simulink model "ev_tms_PID"  (R2023a)
settings: Solver=VariableStepAuto  StartTime=0.0  StopTime=600  FixedStep=1  RelTol=1e-3  AbsTol=1e-3
model workspace: external: MATLAB File /Users/rossschrader/Desktop/ML/ME/_Project/_v3/ev_tms_v3_params.m (data not in the file)
undefined symbols (not defined in the file or in its folder): battery_C1_LUT, battery_capacity_LUT, battery_cell_cp, battery_cell_mass, battery_Em_LUT, battery_N_cells, battery_Qe_init, battery_R0_LUT, battery_R1_LUT, battery_SOC_LUT, battery_T_init, battery_temperature_LUT, bulb, cabin_duct_area, cabin_T_init, chiller_area_primary, chiller_N_baffles, chiller_N_tubes, chiller_tube_D, chiller_tube_L, chiller_wall_conductivity, chiller_wall_thickness, compressor_rpm_LUT, condenser_air_area_flow, condenser_air_area_primary, condenser_W, condenser_wall_conductivity, condenser_wall_thickness, coolant_channel_D, coolant_pipe_D, coolant_T_init, coolant_tank_area, coolant_tank_volume, coolant_valve_D_ratio_max, coolant_valve_D_ratio_min, coolant_valve_displacement, coolant_valve_S_max, evaporator_air_area_flow, evaporator_air_area_primary, evaporator_P_target, evaporator_W, evaporator_wall_conductivity, evaporator_wall_thickness, outlet, pump_speed_max, radiator_air_area_flow, radiator_air_area_primary, radiator_W, radiator_wall_conductivity, radiator_wall_thickness, refrigerant_alpha_init, refrigerant_pipe_D
libraries: fl_lib x221, nesl_utility x79, SimscapeFluids_lib x25, LiBatteryElements_lib x16, sdl_lib x3, slpidlib x2, simulink x1, rllib x1, autolibshared x1, SignalEditorBlockLib x1
(part 5 of 7)

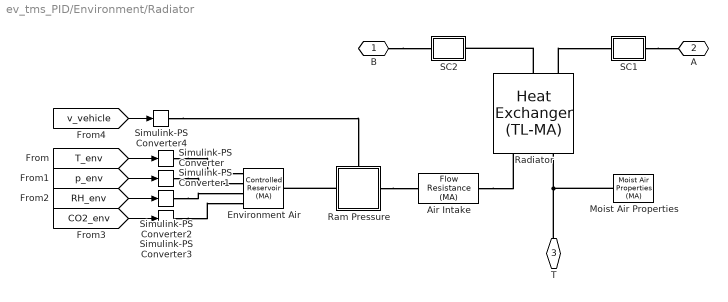
== system ev_tms_PID/Environment/Radiator ==
  Air Intake : fl_lib/Moist Air/Elements/Flow Resistance (MA)  delta_p_nominal=5e-4 MPa  mdot_nominal=1 kg/s  rho_nominal=1.2 kg/m^3  area=cabin_duct_area m^2  laminar_fraction=1e-3
  Environment Air : fl_lib/Moist Air/Elements/Controlled Reservoir (MA)  moisture_spec=foundation.enum.moisture_spec.relative_humidity  trace_gas_spec=foundation.enum.trace_gas_spec.mole_fraction  RH_ws=1  area_A=cabin_duct_area m^2  input_error_spec=foundation.enum.input_range_error.warn
      settings: InternalSimscapePortConfiguration="{\"Bottom\":[],\"Left\":[{\"id\":\"A\",\"label\":\"A\",\"type\":\"foundation.moist_air.moist_air\"}],\"Right\":[{\"id\":\"T\",\"label\":\"T\",\"type\":\"input\"},{\"id\":\"P\",\"label\":\"P\",\"type\":\"input\"},{\"id\":\"W\",\"label\":\"W\",\"type\":\"input\"},{\"id\":\"G\",\"label\":\"G\",\"type\":\"input\"}],\"Top\":[]}"
  Moist Air Properties : fl_lib/Moist Air/Utilities/Moist Air Properties (MA)  R_a=287.047 J/kg/K  T_TLU=[-56.55, -50 : 10 : -10, -5 : 1 : 5, 10 : 10 : 350]' degC  h_a_TLU=[342.416126230579; 349.005511058471; 359.063577249119; 369.119948684177; 379.175469465129; 389.230944678417; 394.258910928084; 395.264534937366; 396.27017101329; 397.275819932805; 398.281482472874; 399.287159410541; 400.292851523015; 401.298559587728; 402.304284382408; 403.310026685143; 404.315787274435; 409.34489180313; 419.404921755863; 429.468036401264; 439.535033154839; 449.606720928652; 459.683919949603; 469.767460521911; 479.858181001348; 489.956925196484; 500.064539372946; 510.181869006204; 520.309755403634; 530.449032296018; 540.60052248087; 550.765034584465; 560.943359995745; 571.136270013102; 581.344513234296; 591.568813210327; 601.809866375885; 612.068340261954; 622.344871990218; 632.640067043998; 642.95449830646; 653.288705353699; 663.643193987949; 674.018435994423; 684.414869104228; 694.832897145098; 705.272890361557; 715.735185886199; 726.220088344236; 736.727870574087; 747.258774447567; 757.813011774199] kJ/kg  mu_a_TLU=[14.2568883320012; 14.6140127728333; 15.1517277055779; 15.6806860159119; 16.2012351072083; 16.7137043125028; 16.9670071730589; 17.017438062815; 17.0677930842452; 17.1180725309876; 17.1682766951315; 17.2184058672268; 17.2684603362935; 17.3184403898301; 17.3683463138234; 17.4181783927569; 17.4679369096204; 17.7156358640698; 18.2056751785154; 18.68879035749; 19.1652344664982; 19.6352478927873; 20.099059103658; 20.5568853601578; 21.0089333871663; 21.4554000014051; 21.8964726992323; 22.3323302062775; 22.7631429910631; 23.1890737447833; 23.6102778293792; 24.0269036959922; 24.4390932757886; 24.8469823450548; 25.2507008663546; 25.6503733074314; 26.0461189394339; 26.4380521159325; 26.8262825340948; 27.2109154792923; 27.5920520543128; 27.969789394274; 28.3442208682439; 28.7154362685068; 29.0835219883356; 29.4485611890712; 29.8106339572472; 30.1698174524429; 30.5261860464955; 30.8798114546565; 31.2307628592324; 31.5791070262086] s*uPa  k_a_TLU=[19.8808489374933; 20.4162454629695; 21.2248743590758; 22.0232452890903; 22.8117314495857; 23.5906913619588; 23.9767075412237; 24.053639990175; 24.1304826682191; 24.2072359051629; 24.2839000294007; 24.3604753679152; 24.4369622462801; 24.5133609886625; 24.5896719178249; 24.6658953551279; 24.7420316205333; 25.1214164701832; 25.8738283029331; 26.6180150229276; 27.3542674377332; 28.0828634735341; 28.8040686837224; 29.5181367785657; 30.2253101618423; 30.9258204644224; 31.6198890677835; 32.3077276126633; 32.9895384896798; 33.6655153099498; 34.33584335461; 35.0007000027879; 35.6602551380254; 36.3146715334901; 36.9641052165342; 37.6087058133173; 38.248616874307; 38.8839761815308; 39.5149160384798; 40.1415635435708; 40.7640408480637; 41.3824653993118; 41.9969501701893; 42.6076038755117; 43.2145311762238; 43.8178328720941; 44.4176060836121; 45.013944423749; 45.6069381602018; 46.1966743687041; 46.783237077953; 47.3667074066625] mW/m/K  p_min=1 kPa  p_max=inf MPa  T_min=-56.55 degC  T_max=350 degC  properties_range_check=simscape.enum.assert.action.error  p_atm=0.101325 MPa  T_atm=20 degC  R_w=461.523 J/kg/K  p_ws_TLU=[1.71168953425982e-06; 3.93770601979424e-06; 1.28411717710344e-05; 3.80051394873809e-05; .00010323902900209; .000259873810798063; .000401741022116384; .000437454836117844; .000476040820618202; .000517704666185737; .000562664883741207; .000611212677444345; .000657088049117899; .000705987905898279; .000758082381149132; .000813549384183233; .000872574861129522; .00122818386934022; .0023392147667769; .00424668834054807; .00738442748706953; .0123512704340234; .0199458019246787; .0312006356960619; .0474147199263783; .0701823607447713; .10141797792131; .143375967241115; .198665399739302; .270259606559999; .361500961984849; .476101381081492; .618139196722055; .792053183687694; 1.0026345688121; 1.25501792086105; 1.55467186826983; 1.90739066433297; 2.31928772772542; 2.79679245576864; 3.34665187151016; 3.97593907083533; 4.69207105435535; 5.5028394740883; 6.41645928168037; 7.4416425436169; 8.58770832955728; 9.86474556030261; 11.2838558865497; 12.8575218898034; 14.6001810568052; 16.5291642526045] MPa  h_w_vap_TLU=[2836.88241275372; 2837.81392500514; 2838.63937175807; 2838.7309929628; 2838.06905313927; 2836.62597341095; 2835.60023952573; 2835.37006381376; 2835.13143158077; 2834.88429145066; 2834.62859062897; 2500.93420564316; 2498.55329907119; 2496.17495082036; 2493.79885912205; 2491.42474723191; 2489.05236104642; 2477.20875029194; 2453.54955988604; 2429.83856603313; 2406.00136954922; 2381.97406342174; 2357.69101156389; 2333.08088387814; 2308.06565480412; 2282.56034405021; 2256.47287422313; 2229.70428017508; 2202.14968030993; 2173.69998896199; 2144.24368406447; 2113.66758247452; 2081.85585110571; 2048.68725710494; 2014.03141249899; 1977.7449923284; 1939.66849592886; 1899.62342931686; 1857.40930169838; 1812.79975416601; 1765.53721731251; 1715.32525772152; 1661.81700477787; 1604.59703745016; 1543.1534616334; 1476.83692476464; 1404.80240352424; 1325.92091736114; 1238.61667822208; 1140.5102987018; 1027.62017777647; 892.733785613825] kJ/kg  h_w_TLU=[2396.55944251649; 2408.68643343608; 2427.1988031141; 2445.702165897; 2464.18429108356; 2482.62529466839; 2491.82135326629; 2493.6580151792; 2495.49372578218; 2497.32843835745; 2499.16210446923; 2500.99462758899; 2502.83092214066; 2504.6665223621; 2506.50140563013; 2508.335548891; 2510.16892865793; 2519.32352241995; 2537.56068088674; 2555.67742615292; 2573.6403223998; 2591.4109179101; 2608.9455037701; 2626.19492016262; 2643.10444358428; 2659.61377634497; 2675.58278696023; 2696.1846256545; 2716.49989553741; 2736.6235210957; 2756.61216047011; 2776.50561773853; 2796.33378922508; 2816.11979583049; 2835.88181423877; 2855.63430574511; 2875.38889327595; 2895.15500577172; 2914.94035964689; 2934.75132290228; 2954.59319330244; 2974.47041285505; 2994.38673458964; 3014.34535328009; 3034.34900867103; 3054.40006755764; 3074.50058946898; 3094.65237953784; 3114.85703128106; 3135.11596137801; 3155.43043805905; 3175.80160435813] kJ/kg  mu_w_TLU=[6.81365662228272; 7.04953750742707; 7.40970098298307; 7.76991278093907; 8.13017290129507; 8.49048134405107; 8.67065368632907; 8.70668960445667; 8.74272600580827; 8.77876289038387; 8.81480025818347; 8.85083810920707; 8.88687644345467; 8.92291526092627; 8.95895456162187; 8.99499434554147; 9.03103461268507; 9.21124319676307; 9.57169660671907; 9.93219833907507; 10.2927483938311; 10.6533467709871; 11.0139934705431; 11.3746884924991; 11.7354318368551; 12.0962235036111; 12.4570634927671; 12.8179518043231; 13.1788884382791; 13.5398733946351; 13.9009066733911; 14.2619882745471; 14.6231181981031; 14.9842964440591; 15.3455230124151; 15.7067979031711; 16.0681211163271; 16.4294926518831; 16.7909125098391; 17.1523806901951; 17.5138971929511; 17.8754620181071; 18.2370751656631; 18.5987366356191; 18.9604464279751; 19.3222045427311; 19.6840109798871; 20.0458657394431; 20.4077688213991; 20.7697202257551; 21.1317199525111; 21.4937680016671] s*uPa  k_w_TLU=[11.46288215976; 11.941997488935; 12.676358586935; 13.414208884935; 14.155548382935; 14.900377080935; 15.274099879935; 15.348949115735; 15.423833243535; 15.498752263335; 15.573706175135; 15.648694978935; 15.723718674735; 15.798777262535; 15.873870742335; 15.948999114135; 16.024162377935; 16.400502076935; 17.155798374935; 17.914583872935; 18.676858570935; 19.442622468935; 20.211875566935; 20.984617864935; 21.760849362935; 22.540570060935; 23.323779958935; 24.110479056935; 24.900667354935; 25.694344852935; 26.491511550935; 27.292167448935; 28.096312546935; 28.903946844935; 29.715070342935; 30.529683040935; 31.347784938935; 32.169376036935; 32.994456334935; 33.823025832935; 34.655084530935; 35.490632428935; 36.329669526935; 37.172195824935; 38.018211322935; 38.867716020935; 39.720709918935; 40.577193016935; 41.437165314935; 42.300626812935; 43.167577510935; 44.038017408935] mW/m/K  D_w=25 mm^2/s  trace_gas_model=foundation.enum.trace_gas_model.track_fraction  R_g=188.923 J/kg/K  h_g_TLU=[439.555216260064; 444.670268200251; 452.538618847003; 460.487124258496; 468.522588768941; 476.649415958793; 480.74798538725; 481.57054318762; 482.394052398751; 483.218514288831; 484.043930029015; 484.870300696555; 485.697627277859; 486.525910671489; 487.355151691079; 488.185351068185; 489.016509455051; 493.186704139431; 501.599194953048; 510.107689961685; 518.711611080182; 527.410026793075; 536.201764778798; 545.085474203452; 554.059675505208; 563.122805485367; 572.27325096919; 581.509373027928; 590.829525105886; 600.232066705818; 609.715373581392; 619.277845178105; 628.917909922924; 638.634028838794; 648.424697859328; 658.288449140109; 668.223851601449; 678.229510889093; 688.304068901113; 698.44620299875; 708.654624994591; 718.928079991818; 729.265345132425; 739.665228299475; 750.126566808087; 760.648226111439; 771.229098541268; 781.868102096908; 792.564179292476; 803.316296068366; 814.123440770426; 824.984623198037] kJ/kg  mu_g_TLU=[10.8921054191698; 11.2215357085649; 11.7233300740382; 12.2234238147811; 12.7215124453467; 13.2173328890673; 13.4643203184773; 13.5136406274989; 13.562934752385; 13.6122025024997; 13.6614436900741; 13.7106581301692; 13.7598456406398; 13.8090060420983; 13.8581391578796; 13.9072448140062; 13.9563228391538; 14.2012926853717; 14.6890687376044; 15.1738428124161; 15.6554929043332; 16.1339159800463; 16.6090257998657; 17.0807510097148; 17.5490334645512; 18.0138267508952; 18.4750948814453; 18.9328111390399; 19.3869570507278; 19.8375214755778; 20.2844997922255; 20.7278931741254; 21.1677079421287; 21.6039549853963; 22.036649242835; 22.4658092382469; 22.8914566632375; 23.3136160026627; 23.7323141980278; 24.1475803447965; 24.5594454200432; 24.9679420372927; 25.3731042257492; 25.774967231431; 26.1735673380029; 26.5689417053362; 26.9611282240413; 27.350165384404; 27.73609215832; 28.118947892972; 28.4987722151178; 28.8756049449796] s*uPa  k_g_TLU=[10.489430678843; 10.9507672150864; 11.666197960308; 12.392559739764; 13.1299519771612; 13.8778409888416; 14.2554325416312; 14.3312274189707; 14.4071122346908; 14.4830860227061; 14.5591478179508; 14.6352966574703; 14.7115315815553; 14.787851634907; 14.8642558678259; 14.9407433374142; 15.0173131087819; 15.401364480906; 16.1751373988038; 16.9558134611595; 17.7432208682398; 18.5366976599676; 19.3360988502003; 20.1412225692689; 20.9517507672929; 21.7672310558863; 22.5871115634685; 23.4107980865695; 24.2377021890869; 25.0672663781241; 25.8989689893876; 26.732318357514; 27.5668446164644; 28.4020933015927; 29.2376215872816; 30.0729965057542; 30.9077942826816; 31.7416001931033; 32.5740086297993; 33.4046232539953; 34.2330571812868; 35.0589331874899; 35.8818839295189; 36.701552179391; 37.5175910702657; 38.3296643536716; 39.1374466671854; 39.9406238119064; 40.7388930391313; 41.5319633456945; 42.3195557774861; 43.1014037407076] mW/m/K  D_g=16 mm^2/s
  Radiator : SimscapeFluids_lib/Fluid Network Interfaces/Heat Exchangers/Heat Exchanger (TL-MA)  flow_arrangement=fluids.interfaces.heat_exchangers.enum.FlowArrangementTLMA.Cross  cross_flow_arrangement=fluids.interfaces.heat_exchangers.enum.CrossFlowArrangementTLMA.MixedUnmixed  R_wall=radiator_wall_thickness / radiator_air_area_primary / radiator_wall_conductivity K/kW  area_A1=pi * coolant_pipe_D^2 / 4 m^2  area_B1=pi * coolant_pipe_D^2 / 4 m^2  area_A2=cabin_duct_area m^2  area_B2=cabin_duct_area m^2  flow_geometry_TL=fluids.interfaces.heat_exchangers.enum.FlowGeometryTL.InsideTubes  tube_num_TL=radiator_N_tubes  tube_length_TL=radiator_L m  tube_cross_section_TL=fluids.interfaces.heat_exchangers.enum.TubeCrossSection.Rectangular  tube_diameter_TL=0.1 m  tube_width_TL=radiator_W m  tube_height_TL=radiator_tube_H m  tube_inner_diameter_TL=0.05 m  tube_outer_diameter_TL=0.1 m  tube_flow_area_TL=0.01 m^2  tube_wetted_perimeter_TL=0.4 m  tube_heat_perimeter_TL=0.4 m  tube_pressure_loss_spec_TL=fluids.interfaces.heat_exchangers.enum.TubePressureLossSpec.Haaland  tube_loss_coeff_TL=10  tube_local_pressure_loss_spec_TL=fluids.thermal_liquid.pipes_fittings.enum.LocalLossSpec.AggregateLength  tube_length_add_TL=radiator_tube_Leq m  tube_local_loss_coefficient_TL=0.1  tube_roughness_pressure_TL=15e-6 m  tube_Re_lam_pressure_TL=2000  tube_Re_tur_pressure_TL=4000  tube_shape_factor_generic_TL=64  tube_heat_coeff_spec_TL=fluids.interfaces.heat_exchangers.enum.TubeHeatCoeffSpec.Gneilinski  tube_colburn_coeff_TL=[.023, .8, .33]  tube_roughness_heat_TL=15e-6 m  tube_Re_lam_heat_TL=2000  tube_Re_tur_heat_TL=4000  tube_Nu_lam_generic_TL=3.66  bank_arrangement_TL=fluids.interfaces.heat_exchangers.enum.BankArrangement.Inline  bank_num_rows_TL=5  bank_tubes_per_row_TL=5  bank_width_TL=1 m  bank_tube_diameter_TL=0.05 m  bank_longitudinal_pitch_TL=0.15 m  bank_transverse_pitch_TL=0.15 m  bank_pressure_loss_spec_TL=fluids.interfaces.heat_exchangers.enum.BankPressureLossSpec.Martin  bank_euler_TL=10  bank_heat_coeff_spec_TL=fluids.interfaces.heat_exchangers.enum.BankHeatCoeffSpec.Martin  bank_colburn_coeff_TL=[.27, .63, .36]  generic_flow_area_TL=0.01 m^2  generic_heat_area_TL=2 m^2  generic_volume_TL=0.05 m^3  generic_loss_coeff_TL=10  generic_colburn_coeff_TL=[.023, .8, .33]  fouling_factor_TL=0.1 m^2*K/kW  fin_area_TL=0 m^2  fin_efficiency_TL=0  p_init_TL=coolant_p_init MPa  T_init_TL=coolant_T_init degC  flow_geometry_MA=fluids.interfaces.heat_exchangers.enum.FlowGeometryMA.Generic  tube_num_MA=1  tube_length_MA=5 m  tube_cross_section_MA=fluids.interfaces.heat_exchangers.enum.TubeCrossSection.Circular  tube_diameter_MA=0.1 m  tube_width_MA=0.1 m  tube_height_MA=0.1 m  tube_inner_diameter_MA=0.05 m  tube_outer_diameter_MA=0.1 m  tube_flow_area_MA=0.01 m^2  tube_wetted_perimeter_MA=0.4 m  tube_heat_perimeter_MA=0.4 m  tube_pressure_loss_spec_MA=fluids.interfaces.heat_exchangers.enum.TubePressureLossSpec.Haaland  tube_loss_coeff_MA=10  tube_local_pressure_loss_spec_MA=fluids.moist_air.pipes_fittings.enum.LocalLossSpec.AggregateLength  tube_length_add_MA=0.1 m  tube_local_loss_coefficient_MA=0.1  tube_roughness_pressure_MA=15e-6 m  tube_Re_lam_pressure_MA=2000  tube_Re_tur_pressure_MA=4000  tube_shape_factor_generic_MA=64  tube_heat_coeff_spec_MA=fluids.interfaces.heat_exchangers.enum.TubeHeatCoeffSpec.Gneilinski  tube_colburn_coeff_MA=[.023, .8, .33]  tube_roughness_heat_MA=15e-6 m  tube_Re_lam_heat_MA=2000  tube_Re_tur_heat_MA=4000  tube_Nu_lam_generic_MA=3.66  bank_arrangement_MA=fluids.interfaces.heat_exchangers.enum.BankArrangement.Inline  bank_num_rows_MA=5  bank_tubes_per_row_MA=5  bank_width_MA=1 m  bank_tube_diameter_MA=0.05 m  bank_longitudinal_pitch_MA=0.15 m  bank_transverse_pitch_MA=0.15 m  bank_pressure_loss_spec_MA=fluids.interfaces.heat_exchangers.enum.BankPressureLossSpec.Martin  bank_euler_MA=10  bank_heat_coeff_spec_MA=fluids.interfaces.heat_exchangers.enum.BankHeatCoeffSpec.Martin  bank_colburn_coeff_MA=[.27, .63, .36]  generic_flow_area_MA=radiator_air_area_flow m^2  generic_heat_area_MA=radiator_air_area_primary m^2  generic_volume_MA=radiator_air_area_flow * radiator_W m^3  generic_loss_coeff_MA=10  generic_colburn_coeff_MA=[0.27, 0.63, 0.36]  fouling_factor_MA=0.1 m^2*K/kW  fin_area_MA=radiator_air_area_fins m^2  fin_efficiency_MA=0.7  p_init_MA=cabin_p_init MPa  T_init_MA=cabin_T_init degC  moisture_spec_MA=foundation.enum.moisture_spec.relative_humidity  RH_init_MA=cabin_RH_init  x_w_init_MA=0.01  y_w_init_MA=0.01  HR_init_MA=0.01  trace_gas_spec_MA=foundation.enum.trace_gas_spec.mole_fraction  x_g_init_MA=0.001  y_g_init_MA=cabin_CO2_init  RH_ws_MA=1
      settings: InternalSimscapePortConfiguration="{\"Bottom\":[],\"Left\":[{\"id\":\"A1\",\"label\":\"A1\",\"type\":\"foundation.thermal_liquid.thermal_liquid\"},{\"id\":\"B1\",\"label\":\"B1\",\"type\":\"foundation.thermal_liquid.thermal_liquid\"}],\"Right\":[{\"id\":\"A2\",\"label\":\"A2\",\"type\":\"foundation.moist_air.moist_air\"},{\"id\":\"B2\",\"label\":\"B2\",\"type\":\"foundation.moist_air.moist_air\"}],\"Top\":[{\"id\":\"W\",\"label\":\"W\",\"type\":\"output\"}]}"
  Ram Pressure : Subsystem
      settings: PortSchema="{\"entries\":[{\"content\":{\"sides\":[{\"content\":{\"connectorIds\":[\"LConn1\"]},\"type\":\"ConnectorPlacement.EquallySpacedRectSide\",\"uuid\":\"75e3029b-49fb-4aa2-a270-5647ec8f7cc2\"},{\"content\":{\"connectorIds\":[\"RConn1\"],\"side\":\"RIGHT\"},\"type\":\"ConnectorPlacement.EquallySpacedRectSide\",\"uuid\":\"a5773782-5ea1-4526-866f-91c4aa99dd69\"},{\"content\":{\"connectorIds\":[\"LConn2\"],\"side\":\"TOP\"},\"type\":\"ConnectorPlacement.EquallySpacedRectSide\",\"uuid\":\"b1426a6c-920c-4fe3-a6f1-49137f31d8b5\"}]},\"type\":\"ConnectorPlacement.EquallySpacedConnector\",\"uuid\":\"8a57436c-822b-4551-8b15-f9c616e1048b\"}],\"packageUris\":[\"http://schema.mathworks.com/mf0/Connector/R2020b\"],\"version\":\"1.0\"}"
  SC1 : Subsystem
      mask Display: disp(get_param(gcb, 'Name'))
  SC2 : Subsystem
      mask Display: disp(get_param(gcb, 'Name'))
  Simulink-PS Converter : nesl_utility/Simulink-PS Converter  PhysicalDomain=network_engine_domain  SubClassName=ps_input  LeftPortType=input  RightPortType=output  PseudoPeriodic=off  Frequencies=[]  NoiseDistribution=none  NoiseParameters=[]  Unit=degC  AffineConversion=on  FilteringAndDerivatives=provide  SimscapeFilterOrder=1  InputFilterTimeConstant=0.001  UdotUserProvided=0
  Simulink-PS Converter1 : nesl_utility/Simulink-PS Converter  PhysicalDomain=network_engine_domain  SubClassName=ps_input  LeftPortType=input  RightPortType=output  PseudoPeriodic=off  Frequencies=[]  NoiseDistribution=none  NoiseParameters=[]  Unit=MPa  AffineConversion=off  FilteringAndDerivatives=provide  SimscapeFilterOrder=1  InputFilterTimeConstant=0.001  UdotUserProvided=0
  Simulink-PS Converter2 : nesl_utility/Simulink-PS Converter  PhysicalDomain=network_engine_domain  SubClassName=ps_input  LeftPortType=input  RightPortType=output  PseudoPeriodic=off  Frequencies=[]  NoiseDistribution=none  NoiseParameters=[]  Unit=1  AffineConversion=off  FilteringAndDerivatives=provide  SimscapeFilterOrder=1  InputFilterTimeConstant=0.001  UdotUserProvided=0
  Simulink-PS Converter3 : nesl_utility/Simulink-PS Converter  PhysicalDomain=network_engine_domain  SubClassName=ps_input  LeftPortType=input  RightPortType=output  PseudoPeriodic=off  Frequencies=[]  NoiseDistribution=none  NoiseParameters=[]  Unit=1  AffineConversion=off  FilteringAndDerivatives=provide  SimscapeFilterOrder=1  InputFilterTimeConstant=0.001  UdotUserProvided=0
  Simulink-PS Converter4 : nesl_utility/Simulink-PS Converter  PhysicalDomain=network_engine_domain  SubClassName=ps_input  LeftPortType=input  RightPortType=output  PseudoPeriodic=off  Frequencies=[]  NoiseDistribution=none  NoiseParameters=[]  Unit=km/hr  AffineConversion=off  FilteringAndDerivatives=provide  SimscapeFilterOrder=1  InputFilterTimeConstant=0.001  UdotUserProvided=0
  B : PMIOPort  Side=Left
  A : PMIOPort  Port=2  Side=Right
  T : PMIOPort  Port=3  Side=Right
  wires:
  [RH_env] -> Simulink-PS Converter2/1
  [CO2_env] -> Simulink-PS Converter3/1
  [T_env] -> Simulink-PS Converter/1
  [p_env] -> Simulink-PS Converter1/1
  [v_vehicle] -> Simulink-PS Converter4/1
  connections:
  B/RConn1 -- SC2/LConn1
  Radiator/LConn1 -- SC1/LConn1
  SC1/RConn1 -- A/RConn1
  Radiator/LConn2 -- SC2/RConn1
  Simulink-PS Converter1/RConn1 -- Environment Air/RConn2
  Simulink-PS Converter2/RConn1 -- Environment Air/RConn3
  Simulink-PS Converter3/RConn1 -- Environment Air/RConn4
  Simulink-PS Converter/RConn1 -- Environment Air/RConn1
  T/RConn1 -- Moist Air Properties/RConn1 -- Radiator/RConn1
  Air Intake/RConn1 -- Radiator/RConn2
  Ram Pressure/RConn1 -- Air Intake/LConn1
  Ram Pressure/LConn1 -- Environment Air/LConn1
  Simulink-PS Converter4/RConn1 -- Ram Pressure/LConn2

== system ev_tms_PID/Environment/Radiator Bypass Valve ==
  Bias : Bias  Bias=-1  SaturateOnIntegerOverflow=off
  Flow Resistance (TL) : fl_lib/Thermal Liquid/Elements/Flow Resistance (TL)  delta_p_nominal=0.001 MPa  mdot_nominal=0.3 kg/s  area=pi * coolant_pipe_D^2 / 4 m^2  laminar_fraction=1e-3
  Gain : Gain  Gain=2
  Max Valve Displacement [m] : Gain  Gain=coolant_valve_displacement
  Radiator Bypass Valve : SimscapeFluids_lib/Thermal Liquid/Valves & Orifices/Directional Control Valves/3-Way Directional Valve (TL)  open_orifices_pos=fluids.thermal_liquid.valves.directional_control_valves.enum.OpenOrifices3Way.PA  open_orifices_neg=fluids.thermal_liquid.valves.directional_control_valves.enum.OpenOrifices3Way.AT  area_spec=fluids.thermal_liquid.valves.directional_control_valves.enum.area_spec.identical  valve_spec=fluids.thermal_liquid.valves.enum.orifice_spec.linear  del_S_max=coolant_valve_displacement m  area_max=pi * (coolant_valve_D_ratio_max*coolant_pipe_D)^2 / 4 m^2  del_S_TLU=[0 0.002 0.004 0.007 0.017] m  valve_area_TLU=[1e-09, 2.0352e-07, 4.0736e-05, .00011438, .00034356] m^2  del_S_flow_TLU=[0 0.002 0.004 0.007 0.017] m  p_diff_TLU=[-.1, .3, .5, .7] MPa  vol_flow_TLU=1e-3 * [1.7e-05, 2e-05, 2.6e-05; .0035, .0045, .0053; .7, .9, 1.06; 1.96, 2.5, 3; 6, 7.7, 9.13] m^3/s  mdot_TLU=[-1e-05, 1.7e-05, 2e-05, 2.6e-05; -.002, .0035, .0045, .0053; -.4, .7, .9, 1.06; -1.13, 1.96, 2.5, 3; -3.45, 6, 7.7, 9.13] kg/s  T_ref_in=293.15 K  p_ref_in=0.101325 MPa  area_leak=pi * (coolant_valve_D_ratio_min*coolant_pipe_D)^2 / 4 m^2  Cd=0.7  Re_c=12  smoothing_factor=0.01  pressure_recovery=simscape.enum.onoff.on  area=pi * coolant_pipe_D^2 / 4 m^2  S_max_PA=coolant_valve_S_max m  del_S_max_PA=coolant_valve_displacement-(coolant_valve_displacement)*(pi * (coolant_valve_D_ratio_min*coolant_pipe_D)^2 / 4)/(pi * (coolant_valve_D_ratio_max*coolant_pipe_D)^2 / 4) m  area_max_PA=pi * (coolant_valve_D_ratio_max*coolant_pipe_D)^2 / 4 m^2  del_S_TLU_PA=[0 0.002 0.004 0.007 0.017] m  valve_area_TLU_PA=[1e-09, 2.0352e-07, 4.0736e-05, .00011438, .00034356] m^2  del_S_flow_TLU_PA=[0 0.002 0.004 0.007 0.017] m  p_diff_TLU_PA=[-.1, .3, .5, .7] MPa  vol_flow_TLU_PA=1e-3 * [1.7e-05, 2e-05, 2.6e-05; .0035, .0045, .0053; .7, .9, 1.06; 1.96, 2.5, 3; 6, 7.7, 9.13] m^3/s  mdot_TLU_PA=[-1e-05, 1.7e-05, 2e-05, 2.6e-05; -.002, .0035, .0045, .0053; -.4, .7, .9, 1.06; -1.13, 1.96, 2.5, 3; -3.45, 6, 7.7, 9.13] kg/s  S_max_AT=-coolant_valve_S_max m  del_S_max_AT=coolant_valve_displacement-(coolant_valve_displacement)*(pi * (coolant_valve_D_ratio_min*coolant_pipe_D)^2 / 4)/(pi * (coolant_valve_D_ratio_max*coolant_pipe_D)^2 / 4) m  area_max_AT=pi * (coolant_valve_D_ratio_max*coolant_pipe_D)^2 / 4 m^2  del_S_TLU_AT=[0 0.002 0.004 0.007 0.017] m  valve_area_TLU_AT=[1e-09, 2.0352e-07, 4.0736e-05, .00011438, .00034356] m^2  del_S_flow_TLU_AT=[0 0.002 0.004 0.007 0.017] m  p_diff_TLU_AT=[-.1, .3, .5, .7] MPa  vol_flow_TLU_AT=1e-3 * [1.7e-05, 2e-05, 2.6e-05; .0035, .0045, .0053; .7, .9, 1.06; 1.96, 2.5, 3; 6, 7.7, 9.13] m^3/s  mdot_TLU_AT=[-1e-05, 1.7e-05, 2e-05, 2.6e-05; -.002, .0035, .0045, .0053; -.4, .7, .9, 1.06; -1.13, 1.96, 2.5, 3; -3.45, 6, 7.7, 9.13] kg/s  S_max_PT=2.5e-3 m  del_S_max_PT=0.005 m  area_max_PT=1e-4 m^2  del_S_TLU_PT=[0, .002, .004, .007, .017] m  valve_area_TLU_PT=[1e-09, 2.0352e-07, 4.0736e-05, .00011438, .00034356] m^2  del_S_flow_TLU_PT=[0, .002, .004, .007, .017] m  p_diff_TLU_PT=[.3, .5, .7] MPa  vol_flow_TLU_PT=1e-3 * [1.7e-05, 2e-05, 2.6e-05; .0035, .0045, .0053; .7, .9, 1.06; 1.96, 2.5, 3; 6, 7.7, 9.13] m^3/s  mdot_TLU_PT=[1.7e-05, 2e-05, 2.6e-05; .0035, .0045, .0053; .7, .9, 1.06; 1.96, 2.5, 3; 6, 7.7, 9.13] kg/s
      settings: InternalSimscapePortConfiguration="{\"Bottom\":[],\"Left\":[{\"id\":\"A\",\"label\":\"A\",\"type\":\"foundation.thermal_liquid.thermal_liquid\"}],\"Right\":[{\"id\":\"S\",\"label\":\"S\",\"type\":\"input\"},{\"id\":\"P\",\"label\":\"P\",\"type\":\"foundation.thermal_liquid.thermal_liquid\"},{\"id\":\"T\",\"label\":\"T\",\"type\":\"foundation.thermal_liquid.thermal_liquid\"}],\"Top\":[]}"
  Simulink-PS Converter : nesl_utility/Simulink-PS Converter  PhysicalDomain=network_engine_domain  SubClassName=ps_input  LeftPortType=input  RightPortType=output  PseudoPeriodic=off  Frequencies=[]  NoiseDistribution=none  NoiseParameters=[]  Unit=m  AffineConversion=off  FilteringAndDerivatives=provide  SimscapeFilterOrder=1  InputFilterTimeConstant=0.001  UdotUserProvided=0
  Transfer Fcn : TransferFcn  Denominator=[1 1]
  B : PMIOPort  Side=Left
  C : PMIOPort  Port=2  Side=Left
  A : PMIOPort  Port=3  Side=Right
  wires:
  Max Valve Displacement [m]/1 -> Simulink-PS Converter/1
  Bias/1 -> Max Valve Displacement [m]/1
  Gain/1 -> Bias/1
  [cmd_rad_bypass] -> Transfer Fcn/1
  Transfer Fcn/1 -> Gain/1
  connections:
  Radiator Bypass Valve/LConn1 -- A/RConn1
  Radiator Bypass Valve/RConn3 -- C/RConn1
  Radiator Bypass Valve/RConn1 -- Simulink-PS Converter/RConn1
  B/RConn1 -- Flow Resistance (TL)/RConn1
  Radiator Bypass Valve/RConn2 -- Flow Resistance (TL)/LConn1

== system ev_tms_PID/Reward/Power Reward ==
  Add : Sum  Commented=on  Inputs=7
  From : From  Commented=on  GotoTag=motor_pump_pwr  TagVisibility=global
  From1 : From  Commented=on  GotoTag=bat_pump_pwr  TagVisibility=global
  From2 : From  Commented=on  GotoTag=fan_pwr  TagVisibility=global
  From3 : From  Commented=on  GotoTag=compressor_pwr  TagVisibility=global
  From4 : From  Commented=on  GotoTag=blower_pwr  TagVisibility=global
  From5 : From  Commented=on  GotoTag=PTC_pwr  TagVisibility=global
  From6 : From  Commented=on  GotoTag=heater_pwr  TagVisibility=global
  Gain : Gain  Commented=on  Gain=-.01
  Gain1 : Gain  Gain=-.05
  Power : Outport
  wires:
  From/1 -> Add/1
  From1/1 -> Add/2
  From2/1 -> Add/3
  From3/1 -> Add/4
  From4/1 -> Add/5
  From5/1 -> Add/6
  From6/1 -> Add/7
  Add/1 -> Gain/1
  [blower_pwr] -> Gain1/1
  Gain1/1 -> Power/1

== system ev_tms_PID/Reward/Temp Reward ==
  note: T cabin Reward
  Abs : Abs  SaturateOnIntegerOverflow=off
  Add1 : Sum  Inputs=+-
  If Action Subsystem11 : Subsystem  TreatAsAtomicUnit=on
  If Action Subsystem9 : Subsystem  TreatAsAtomicUnit=on
  If3 : If  IfExpression=u1 > 0.5  ZeroCross=off
  Merge3 : Merge
  Temp : Outport
  wires:
  Abs/1 -> If Action Subsystem9/1(Input), If3/1
  Add1/1 -> Abs/1
  [T_cabin] -> Add1/1
  Merge3/1 -> Temp/1
  If Action Subsystem9/1(Out1) -> Merge3/1
  [T_setpoint] -> Add1/2
  If3/2 -> If Action Subsystem11/Action
  If3/1 -> If Action Subsystem9/Action
  If Action Subsystem11/1(Out1) -> Merge3/2

== system ev_tms_PID/Reward1/Power Reward ==
  Add : Sum  Commented=on  Inputs=7
  From : From  Commented=on  GotoTag=motor_pump_pwr  TagVisibility=global
  From1 : From  Commented=on  GotoTag=bat_pump_pwr  TagVisibility=global
  From2 : From  Commented=on  GotoTag=fan_pwr  TagVisibility=global
  From3 : From  Commented=on  GotoTag=compressor_pwr  TagVisibility=global
  From4 : From  Commented=on  GotoTag=blower_pwr  TagVisibility=global
  From5 : From  Commented=on  GotoTag=PTC_pwr  TagVisibility=global
  From6 : From  Commented=on  GotoTag=heater_pwr  TagVisibility=global
  Gain : Gain  Commented=on  Gain=-.01
  Gain1 : Gain  Gain=-.05
  Power : Outport
  wires:
  From/1 -> Add/1
  From1/1 -> Add/2
  From2/1 -> Add/3
  From3/1 -> Add/4
  From4/1 -> Add/5
  From5/1 -> Add/6
  From6/1 -> Add/7
  Add/1 -> Gain/1
  [blower_pwr] -> Gain1/1
  Gain1/1 -> Power/1

== system ev_tms_PID/Reward1/Temp Reward ==
  note: T cabin Reward
  Abs : Abs  SaturateOnIntegerOverflow=off
  Add1 : Sum  Inputs=+-
  If Action Subsystem11 : Subsystem  TreatAsAtomicUnit=on
  If Action Subsystem9 : Subsystem  TreatAsAtomicUnit=on
  If3 : If  IfExpression=u1 > 0.5  ZeroCross=off
  Merge3 : Merge
  Temp : Outport
  wires:
  Abs/1 -> If Action Subsystem9/1(Input), If3/1
  Add1/1 -> Abs/1
  [T_cabin] -> Add1/1
  Merge3/1 -> Temp/1
  If Action Subsystem9/1(Out1) -> Merge3/1
  [T_setpoint] -> Add1/2
  If3/2 -> If Action Subsystem11/Action
  If3/1 -> If Action Subsystem9/Action
  If Action Subsystem11/1(Out1) -> Merge3/2

== system ev_tms_PID/Scenario/Power Demand ==
  speed : Inport
  Charger Heat vs Current : Lookup_n-D  NumberOfTableDimensions=1  BreakpointsForDimension1=[-100 0 25 50 300]  IndexSearchMethod=Linear search  BeginIndexSearchUsingPreviousIndexResult=on  Table=[250 0 40 70 400]  InternalRulePriority=Speed  RndMeth=Simplest
  DCDC Heat vs Current : Lookup_n-D  NumberOfTableDimensions=1  BreakpointsForDimension1=[-100 0 25 50 300]  IndexSearchMethod=Linear search  BeginIndexSearchUsingPreviousIndexResult=on  Table=[250 0 40 70 400]  InternalRulePriority=Speed  RndMeth=Simplest
  Derivative : Subsystem  mask(1-st Order Filter Derivative){tau=1}
      mask prompts: tau "Filter time constant [s]"
  Inverter Current vs Acceleration : Lookup_n-D  NumberOfTableDimensions=1  BreakpointsForDimension1=[-10 -8 -5 0 5 8 10]  IndexSearchMethod=Linear search  BeginIndexSearchUsingPreviousIndexResult=on  Table=[200 150 100 0 100 150 200]*0.6  InternalRulePriority=Speed  RndMeth=Simplest
  Inverter Current vs Speed : Lookup_n-D  NumberOfTableDimensions=1  BreakpointsForDimension1=[0 60 80 100 120 140 160 180 200]  IndexSearchMethod=Linear search  BeginIndexSearchUsingPreviousIndexResult=on  Table=[0 10 18 27 45 65 100 120 160]  InternalRulePriority=Speed  RndMeth=Simplest
  Inverter Heat vs Current : Lookup_n-D  NumberOfTableDimensions=1  BreakpointsForDimension1=[-100 0 25 50 300]  IndexSearchMethod=Linear search  BeginIndexSearchUsingPreviousIndexResult=on  Table=[250 0 40 70 400]  InternalRulePriority=Speed  RndMeth=Simplest
  Motor Heat vs Current : Lookup_n-D  NumberOfTableDimensions=1  BreakpointsForDimension1=[-150 -70 -26 0 25 50 100 300 600]  IndexSearchMethod=Linear search  BeginIndexSearchUsingPreviousIndexResult=on  Table=[3500 2650 2100 0 400 550 4800 4800 4800]  InternalRulePriority=Speed  RndMeth=Simplest
  Saturation : Saturate  UpperLimit=200  LowerLimit=-inf
  Sum : Sum  Inputs=|++
  Transfer Fcn{,1..4} (5 alike) : TransferFcn  Denominator=[1 1]
  I_battery : Outport
  Q_inverter : Outport  Port=2
  Q_motor : Outport  Port=3
  Q_charger : Outport  Port=4
  Q_dcdc : Outport  Port=5
  wires:
  Derivative/1(A) -> Inverter Current vs Acceleration/1
  speed/1 -> Inverter Current vs Speed/1, Derivative/1(V)
  Inverter Current vs Speed/1 -> Sum/1
  Inverter Current vs Acceleration/1 -> Sum/2
  Sum/1 -> Saturation/1
  Saturation/1 -> Inverter Heat vs Current/1, Motor Heat vs Current/1, DCDC Heat vs Current/1, Charger Heat vs Current/1, Transfer Fcn/1
  Inverter Heat vs Current/1 -> Transfer Fcn1/1
  Motor Heat vs Current/1 -> Transfer Fcn2/1
  Charger Heat vs Current/1 -> Transfer Fcn3/1
  Transfer Fcn/1 -> I_battery/1
  Transfer Fcn1/1 -> Q_inverter/1
  Transfer Fcn2/1 -> Q_motor/1
  Transfer Fcn3/1 -> Q_charger/1
  DCDC Heat vs Current/1 -> Transfer Fcn4/1
  Transfer Fcn4/1 -> Q_dcdc/1

== system ev_tms_PID/Controls/Coolant Loop Control/Battery Heater ==
  T_env : Inport
  T_coolant_battery_in : Inport  Port=2
  Constant : Constant  Value=0
  Relay : Relay  OnSwitchValue=15  OffSwitchValue=5  OnOutputValue=0  OffOutputValue=1  ZeroCross=off
  Switch : Switch  Criteria=u2 > Threshold  Threshold=5  SaturateOnIntegerOverflow=off  InputSameDT=off
  cmd_heater : Outport
  wires:
  T_coolant_battery_in/1 -> Relay/1
  Switch/1 -> cmd_heater/1
  T_env/1 -> Switch/2
  Relay/1 -> Switch/3
  Constant/1 -> Switch/1

== system ev_tms_PID/Controls/Coolant Loop Control/Battery Pump ==
  cmd_motor_pump : Inport
  T_battery : Inport  Port=2
  cmd_chiller_bypass : Inport  Port=3
  parallel_serial : Inport  Port=4
  Constant : Constant  Value=0.3
  Constant1 : Constant  Value=0.5
  MinMax : MinMax  Function=max  Inputs=2
  Relay : Relay  OnSwitchValue=50  OffSwitchValue=45
  Switch : Switch  Criteria=u2 > Threshold  Threshold=0.5  SaturateOnIntegerOverflow=off  InputSameDT=off
  Switch1 : Switch  Criteria=u2 > Threshold  Threshold=0.5  SaturateOnIntegerOverflow=off  InputSameDT=off
  cmd_battery_pump : Outport
  wires:
  T_battery/1 -> Relay/1
  parallel_serial/1 -> Switch/2
  Switch/1 -> cmd_battery_pump/1
  Constant/1 -> Switch1/1
  Constant1/1 -> Switch1/3
  cmd_chiller_bypass/1 -> Switch1/2
  Relay/1 -> MinMax/1
  Switch1/1 -> MinMax/2
  MinMax/1 -> Switch/3
  cmd_motor_pump/1 -> Switch/1

== system ev_tms_PID/Controls/Coolant Loop Control/Chiller Bypass ==
  T_battery : Inport
  Relay : Relay  OnSwitchValue=35  OffSwitchValue=30  OnOutputValue=0  OffOutputValue=1
  cmd_chiller_bypass : Outport
  wires:
  Relay/1 -> cmd_chiller_bypass/1
  T_battery/1 -> Relay/1

== system ev_tms_PID/Controls/Coolant Loop Control/Motor Pump ==
  T_motor : Inport
  1-D Lookup Table : Lookup_n-D  NumberOfTableDimensions=1  BreakpointsForDimension1=[-50 45 48 52 58 60 75 130]  IndexSearchMethod=Linear search  BeginIndexSearchUsingPreviousIndexResult=on  Table=[0 0 0.1 0.3 0.5 0.7 1 1]  InternalRulePriority=Speed  RndMeth=Simplest
  Saturation : Saturate  UpperLimit=1  LowerLimit=0.3
  cmd_motor_pump : Outport
  wires:
  T_motor/1 -> 1-D Lookup Table/1
  1-D Lookup Table/1 -> Saturation/1
  Saturation/1 -> cmd_motor_pump/1

== system ev_tms_PID/Controls/Coolant Loop Control/Parallel-Serial Mode ==
  note: 0 = Parallel mode
      |
      | 1 = Serial mode
  cmd_chiller_bypass : Inport
  T_env : Inport  Port=2
  T_coolant_inverter_out : Inport  Port=3
  Constant : Constant  Value=0
  MinMax : MinMax  Function=max  Inputs=2
  Relay : Relay  OnSwitchValue=35  OffSwitchValue=30  OnOutputValue=0  OffOutputValue=1
  Switch : Switch  Criteria=u2 > Threshold  Threshold=0.5  SaturateOnIntegerOverflow=off  InputSameDT=off
  cmd_parallel_serial : Outport
  wires:
  T_env/1 -> MinMax/1
  T_coolant_inverter_out/1 -> MinMax/2
  MinMax/1 -> Relay/1
  Constant/1 -> Switch/3
  Switch/1 -> cmd_parallel_serial/1
  cmd_chiller_bypass/1 -> Switch/2
  Relay/1 -> Switch/1

== system ev_tms_PID/Controls/Coolant Loop Control/Radiator Bypass ==
  T_coolant_inverter_out : Inport
  Relay : Relay  OnSwitchValue=25  OffSwitchValue=20  OnOutputValue=0  OffOutputValue=1
  cmd_rad_bypass : Outport
  wires:
  Relay/1 -> cmd_rad_bypass/1
  T_coolant_inverter_out/1 -> Relay/1

== system ev_tms_PID/Controls/Fan Control/Condenser Requirement ==
  p_cond : Inport
  T_env : Inport  Port=2
  1-D Lookup Table : Lookup_n-D  NumberOfTableDimensions=1  BreakpointsForDimension1=[0 20 30 40 50]  IndexSearchMethod=Linear search  BeginIndexSearchUsingPreviousIndexResult=on  Table=[2.0 2.0 1.8 1.5 1.3]  InternalRulePriority=Speed  RndMeth=Simplest
  1-D Lookup Table1 : Lookup_n-D  NumberOfTableDimensions=1  BreakpointsForDimension1=[0 20 30 40 50]  IndexSearchMethod=Linear search  BeginIndexSearchUsingPreviousIndexResult=on  Table=[1.4 1.4 1.3 1.2 1.1]  InternalRulePriority=Speed  RndMeth=Simplest
  1-D Lookup Table2 : Lookup_n-D  NumberOfTableDimensions=1  BreakpointsForDimension1=[0 20 30 40 50]  IndexSearchMethod=Linear search  BeginIndexSearchUsingPreviousIndexResult=on  Table=[0.8 0.8 0.8 0.8 0.8]  InternalRulePriority=Speed  RndMeth=Simplest
  Bias : Bias  Bias=0.4  SaturateOnIntegerOverflow=off
  Bias1 : Bias  Bias=0.4  SaturateOnIntegerOverflow=off
  Bias2 : Bias  Bias=0.3  SaturateOnIntegerOverflow=off
  Gain : Gain  Gain=1/3
  Relay Level 1 : Subsystem
  Relay Level 2 : Subsystem
  Relay Level 3 : Subsystem
  Sum : Sum  Inputs=+++
  cmd_fan : Outport
  wires:
  Sum/1 -> Gain/1
  p_cond/1 -> Relay Level 3/1(in), Relay Level 2/1(in), Relay Level 1/1(in)
  Relay Level 3/1(out) -> Sum/1
  Relay Level 2/1(out) -> Sum/2
  Relay Level 1/1(out) -> Sum/3
  1-D Lookup Table/1 -> Relay Level 3/3(low), Bias/1
  Bias/1 -> Relay Level 3/2(high)
  1-D Lookup Table1/1 -> Relay Level 2/3(low), Bias1/1
  Bias1/1 -> Relay Level 2/2(high)
  1-D Lookup Table2/1 -> Relay Level 1/3(low), Bias2/1
  Bias2/1 -> Relay Level 1/2(high)
  T_env/1 -> 1-D Lookup Table/1, 1-D Lookup Table1/1, 1-D Lookup Table2/1
  Gain/1 -> cmd_fan/1

== system ev_tms_PID/Controls/Fan Control/Inverter Requirement ==
  T_inverter : Inport
  Gain : Gain  Gain=1/3
  Relay Level 1 : Relay  OnSwitchValue=75  OffSwitchValue=65
  Relay Level 2 : Relay  OnSwitchValue=85  OffSwitchValue=76
  Relay Level 3 : Relay  OnSwitchValue=95  OffSwitchValue=86
  Sum : Sum  Inputs=+++
  cmd_fan : Outport
  wires:
  T_inverter/1 -> Relay Level 1/1, Relay Level 3/1, Relay Level 2/1
  Relay Level 2/1 -> Sum/2
  Relay Level 3/1 -> Sum/1
  Relay Level 1/1 -> Sum/3
  Sum/1 -> Gain/1
  Gain/1 -> cmd_fan/1

== system ev_tms_PID/Controls/Fan Control/Motor Requirement ==
  T_motor : Inport
  1-D Lookup Table : Lookup_n-D  NumberOfTableDimensions=1  BreakpointsForDimension1=[-50 45 48 52 58 60 75 130]  IndexSearchMethod=Linear search  BeginIndexSearchUsingPreviousIndexResult=on  Table=[0 0 0.1 0.3 0.5 0.7 1 1]  InternalRulePriority=Speed  RndMeth=Simplest
  cmd_fan : Outport
  wires:
  T_motor/1 -> 1-D Lookup Table/1
  1-D Lookup Table/1 -> cmd_fan/1

== system ev_tms_PID/Environment/Battery/Pack 1 ==
  note: Scale up voltage drop
      | to total of N cells
  Controlled Voltage Source : fl_lib/Electrical/Electrical Sources/Controlled Voltage Source
  Lithium Cell 1RC : Subsystem
      settings: PortSchema="{\"entries\":[{\"content\":{\"sides\":[{\"content\":{\"connectorIds\":[]},\"type\":\"ConnectorPlacement.EquallySpacedRectSide\",\"uuid\":\"ccb9f794-c2a7-49a2-9836-26607ca18a9f\"},{\"content\":{\"connectorIds\":[],\"side\":\"RIGHT\"},\"type\":\"ConnectorPlacement.EquallySpacedRectSide\",\"uuid\":\"f1620ab9-2b03-42d4-871e-d35b8093f316\"},{\"content\":{\"connectorIds\":[\"LConn1\",\"LConn2\"],\"side\":\"TOP\"},\"type\":\"ConnectorPlacement.EquallySpacedRectSide\",\"uuid\":\"e679b0d8-ccbe-4539-8d6b-f3ffcd05b92b\"},{\"content\":{\"connectorIds\":[\"RConn1\",\"RConn2\"],\"side\":\"BOTTOM\"},\"type\":\"ConnectorPlacement.EquallySpacedRectSide\",\"uuid\":\"2833ed9d-c0e8-49c1-ad7b-8d4bc87d1df9\"},{\"content\":{\"connectorIds\":[],\"side\":\"HIDDEN\"},\"type\":\"ConnectorPlacement.EquallySpacedRectSide\",\"uuid\":\"76338804-e613-4140-a6be-ae9642a12407\"}]},\"type\":\"ConnectorPlacement.EquallySpacedConnector\",\"uuid\":\"276130fc-4c62-4f99-ae12-f3121ff878f4\"}],\"packageUris\":[\"http://schema.mathworks.com/mf0/Connector/R2020b\"],\"version\":\"1.0\"}"
      mask Display:
      | % Battery icon
      | plot([0 0 0.8 0.8], [0.2 0.9 0.9 1.5])
      | plot([0 0 0.8 0.8], -[0.2 0.9 0.9 1.5])
      | patch([-0.4 0.4 0.4 -0.4], [-0.45 -0.45 -0.15 -0.15], [0 0 0])
      | patch([-0.9 0.9 0.9 -0.9], [0.15 0.15 0.45 0.45], [0 0 0])
      | 
      | % Plot points to set plot range
      | color('white')
      | plot(1.5,1.5)
      | plot(-1.5,-1.5)
      | 
      | % Port labels
      | color('red')
      | port_label('LConn',1,'P')
      | port_label('LConn',2,'+')
      | port_label('RConn',1,'T')
      | port_label('RConn',2,'-')
  N : fl_lib/Physical Signals/Functions/PS Gain  gain=Ncells
  N-1 : fl_lib/Physical Signals/Functions/PS Gain  gain=Ncells - 1
  Thermal Model : Subsystem
  Voltage Sensor : fl_lib/Electrical/Electrical Sensors/Voltage Sensor
  - : PMIOPort  Side=Right
  H : PMIOPort  Port=2  Side=Left
  + : PMIOPort  Port=3  Side=Left
  connections:
  N/RConn1 -- Thermal Model/LConn2
  H/RConn1 -- Thermal Model/LConn1
  -/RConn1 -- Controlled Voltage Source/RConn2
  N-1/RConn1 -- Controlled Voltage Source/RConn1
  +/RConn1 -- Lithium Cell 1RC/LConn2 -- Voltage Sensor/LConn1
  Voltage Sensor/RConn1 -- N-1/LConn1
  Lithium Cell 1RC/RConn2 -- Voltage Sensor/RConn2 -- Controlled Voltage Source/LConn1
  Lithium Cell 1RC/RConn1 -- Thermal Model/RConn1
  Lithium Cell 1RC/LConn1 -- N/LConn1

== system ev_tms_PID/Environment/Battery/Pack 2 ==
  note: Scale up voltage drop
      | to total of N cells
  Controlled Voltage Source : fl_lib/Electrical/Electrical Sources/Controlled Voltage Source
  Lithium Cell 1RC : Subsystem
      settings: PortSchema="{\"entries\":[{\"content\":{\"sides\":[{\"content\":{\"connectorIds\":[]},\"type\":\"ConnectorPlacement.EquallySpacedRectSide\",\"uuid\":\"ccb9f794-c2a7-49a2-9836-26607ca18a9f\"},{\"content\":{\"connectorIds\":[],\"side\":\"RIGHT\"},\"type\":\"ConnectorPlacement.EquallySpacedRectSide\",\"uuid\":\"f1620ab9-2b03-42d4-871e-d35b8093f316\"},{\"content\":{\"connectorIds\":[\"LConn1\",\"LConn2\"],\"side\":\"TOP\"},\"type\":\"ConnectorPlacement.EquallySpacedRectSide\",\"uuid\":\"e679b0d8-ccbe-4539-8d6b-f3ffcd05b92b\"},{\"content\":{\"connectorIds\":[\"RConn1\",\"RConn2\"],\"side\":\"BOTTOM\"},\"type\":\"ConnectorPlacement.EquallySpacedRectSide\",\"uuid\":\"2833ed9d-c0e8-49c1-ad7b-8d4bc87d1df9\"},{\"content\":{\"connectorIds\":[],\"side\":\"HIDDEN\"},\"type\":\"ConnectorPlacement.EquallySpacedRectSide\",\"uuid\":\"76338804-e613-4140-a6be-ae9642a12407\"}]},\"type\":\"ConnectorPlacement.EquallySpacedConnector\",\"uuid\":\"276130fc-4c62-4f99-ae12-f3121ff878f4\"}],\"packageUris\":[\"http://schema.mathworks.com/mf0/Connector/R2020b\"],\"version\":\"1.0\"}"
      mask Display:
      | % Battery icon
      | plot([0 0 0.8 0.8], [0.2 0.9 0.9 1.5])
      | plot([0 0 0.8 0.8], -[0.2 0.9 0.9 1.5])
      | patch([-0.4 0.4 0.4 -0.4], [-0.45 -0.45 -0.15 -0.15], [0 0 0])
      | patch([-0.9 0.9 0.9 -0.9], [0.15 0.15 0.45 0.45], [0 0 0])
      | 
      | % Plot points to set plot range
      | color('white')
      | plot(1.5,1.5)
      | plot(-1.5,-1.5)
      | 
      | % Port labels
      | color('red')
      | port_label('LConn',1,'P')
      | port_label('LConn',2,'+')
      | port_label('RConn',1,'T')
      | port_label('RConn',2,'-')
  N : fl_lib/Physical Signals/Functions/PS Gain  gain=Ncells
  N-1 : fl_lib/Physical Signals/Functions/PS Gain  gain=Ncells - 1
  Thermal Model : Subsystem
  Voltage Sensor : fl_lib/Electrical/Electrical Sensors/Voltage Sensor
  - : PMIOPort  Side=Right
  H : PMIOPort  Port=2  Side=Left
  + : PMIOPort  Port=3  Side=Left
  connections:
  N/RConn1 -- Thermal Model/LConn2
  H/RConn1 -- Thermal Model/LConn1
  -/RConn1 -- Controlled Voltage Source/RConn2
  N-1/RConn1 -- Controlled Voltage Source/RConn1
  +/RConn1 -- Lithium Cell 1RC/LConn2 -- Voltage Sensor/LConn1
  Voltage Sensor/RConn1 -- N-1/LConn1
  Lithium Cell 1RC/RConn2 -- Voltage Sensor/RConn2 -- Controlled Voltage Source/LConn1
  Lithium Cell 1RC/RConn1 -- Thermal Model/RConn1
  Lithium Cell 1RC/LConn1 -- N/LConn1

== system ev_tms_PID/Environment/Battery/Pack 3 ==
  note: Scale up voltage drop
      | to total of N cells
  Controlled Voltage Source : fl_lib/Electrical/Electrical Sources/Controlled Voltage Source
  Lithium Cell 1RC : Subsystem
      settings: PortSchema="{\"entries\":[{\"content\":{\"sides\":[{\"content\":{\"connectorIds\":[]},\"type\":\"ConnectorPlacement.EquallySpacedRectSide\",\"uuid\":\"ccb9f794-c2a7-49a2-9836-26607ca18a9f\"},{\"content\":{\"connectorIds\":[],\"side\":\"RIGHT\"},\"type\":\"ConnectorPlacement.EquallySpacedRectSide\",\"uuid\":\"f1620ab9-2b03-42d4-871e-d35b8093f316\"},{\"content\":{\"connectorIds\":[\"LConn1\",\"LConn2\"],\"side\":\"TOP\"},\"type\":\"ConnectorPlacement.EquallySpacedRectSide\",\"uuid\":\"e679b0d8-ccbe-4539-8d6b-f3ffcd05b92b\"},{\"content\":{\"connectorIds\":[\"RConn1\",\"RConn2\"],\"side\":\"BOTTOM\"},\"type\":\"ConnectorPlacement.EquallySpacedRectSide\",\"uuid\":\"2833ed9d-c0e8-49c1-ad7b-8d4bc87d1df9\"},{\"content\":{\"connectorIds\":[],\"side\":\"HIDDEN\"},\"type\":\"ConnectorPlacement.EquallySpacedRectSide\",\"uuid\":\"76338804-e613-4140-a6be-ae9642a12407\"}]},\"type\":\"ConnectorPlacement.EquallySpacedConnector\",\"uuid\":\"276130fc-4c62-4f99-ae12-f3121ff878f4\"}],\"packageUris\":[\"http://schema.mathworks.com/mf0/Connector/R2020b\"],\"version\":\"1.0\"}"
      mask Display:
      | % Battery icon
      | plot([0 0 0.8 0.8], [0.2 0.9 0.9 1.5])
      | plot([0 0 0.8 0.8], -[0.2 0.9 0.9 1.5])
      | patch([-0.4 0.4 0.4 -0.4], [-0.45 -0.45 -0.15 -0.15], [0 0 0])
      | patch([-0.9 0.9 0.9 -0.9], [0.15 0.15 0.45 0.45], [0 0 0])
      | 
      | % Plot points to set plot range
      | color('white')
      | plot(1.5,1.5)
      | plot(-1.5,-1.5)
      | 
      | % Port labels
      | color('red')
      | port_label('LConn',1,'P')
      | port_label('LConn',2,'+')
      | port_label('RConn',1,'T')
      | port_label('RConn',2,'-')
  N : fl_lib/Physical Signals/Functions/PS Gain  gain=Ncells
  N-1 : fl_lib/Physical Signals/Functions/PS Gain  gain=Ncells - 1
  Thermal Model : Subsystem
  Voltage Sensor : fl_lib/Electrical/Electrical Sensors/Voltage Sensor
  - : PMIOPort  Side=Right
  H : PMIOPort  Port=2  Side=Left
  + : PMIOPort  Port=3  Side=Left
  connections:
  Lithium Cell 1RC/LConn1 -- N/LConn1
  Lithium Cell 1RC/RConn1 -- Thermal Model/RConn1
  Controlled Voltage Source/LConn1 -- Voltage Sensor/RConn2 -- Lithium Cell 1RC/RConn2
  Voltage Sensor/RConn1 -- N-1/LConn1
  Voltage Sensor/LConn1 -- Lithium Cell 1RC/LConn2 -- +/RConn1
  N-1/RConn1 -- Controlled Voltage Source/RConn1
  -/RConn1 -- Controlled Voltage Source/RConn2
  H/RConn1 -- Thermal Model/LConn1
  N/RConn1 -- Thermal Model/LConn2

== system ev_tms_PID/Environment/Battery/Pack 4 ==
  note: Scale up voltage drop
      | to total of N cells
  Controlled Voltage Source : fl_lib/Electrical/Electrical Sources/Controlled Voltage Source
  Lithium Cell 1RC : Subsystem
      settings: PortSchema="{\"entries\":[{\"content\":{\"sides\":[{\"content\":{\"connectorIds\":[]},\"type\":\"ConnectorPlacement.EquallySpacedRectSide\",\"uuid\":\"ccb9f794-c2a7-49a2-9836-26607ca18a9f\"},{\"content\":{\"connectorIds\":[],\"side\":\"RIGHT\"},\"type\":\"ConnectorPlacement.EquallySpacedRectSide\",\"uuid\":\"f1620ab9-2b03-42d4-871e-d35b8093f316\"},{\"content\":{\"connectorIds\":[\"LConn1\",\"LConn2\"],\"side\":\"TOP\"},\"type\":\"ConnectorPlacement.EquallySpacedRectSide\",\"uuid\":\"e679b0d8-ccbe-4539-8d6b-f3ffcd05b92b\"},{\"content\":{\"connectorIds\":[\"RConn1\",\"RConn2\"],\"side\":\"BOTTOM\"},\"type\":\"ConnectorPlacement.EquallySpacedRectSide\",\"uuid\":\"2833ed9d-c0e8-49c1-ad7b-8d4bc87d1df9\"},{\"content\":{\"connectorIds\":[],\"side\":\"HIDDEN\"},\"type\":\"ConnectorPlacement.EquallySpacedRectSide\",\"uuid\":\"76338804-e613-4140-a6be-ae9642a12407\"}]},\"type\":\"ConnectorPlacement.EquallySpacedConnector\",\"uuid\":\"276130fc-4c62-4f99-ae12-f3121ff878f4\"}],\"packageUris\":[\"http://schema.mathworks.com/mf0/Connector/R2020b\"],\"version\":\"1.0\"}"
      mask Display:
      | % Battery icon
      | plot([0 0 0.8 0.8], [0.2 0.9 0.9 1.5])
      | plot([0 0 0.8 0.8], -[0.2 0.9 0.9 1.5])
      | patch([-0.4 0.4 0.4 -0.4], [-0.45 -0.45 -0.15 -0.15], [0 0 0])
      | patch([-0.9 0.9 0.9 -0.9], [0.15 0.15 0.45 0.45], [0 0 0])
      | 
      | % Plot points to set plot range
      | color('white')
      | plot(1.5,1.5)
      | plot(-1.5,-1.5)
      | 
      | % Port labels
      | color('red')
      | port_label('LConn',1,'P')
      | port_label('LConn',2,'+')
      | port_label('RConn',1,'T')
      | port_label('RConn',2,'-')
  N : fl_lib/Physical Signals/Functions/PS Gain  gain=Ncells
  N-1 : fl_lib/Physical Signals/Functions/PS Gain  gain=Ncells - 1
  Thermal Model : Subsystem
  Voltage Sensor : fl_lib/Electrical/Electrical Sensors/Voltage Sensor
  - : PMIOPort  Side=Right
  H : PMIOPort  Port=2  Side=Left
  + : PMIOPort  Port=3  Side=Left
  connections:
  N/RConn1 -- Thermal Model/LConn2
  H/RConn1 -- Thermal Model/LConn1
  -/RConn1 -- Controlled Voltage Source/RConn2
  N-1/RConn1 -- Controlled Voltage Source/RConn1
  +/RConn1 -- Lithium Cell 1RC/LConn2 -- Voltage Sensor/LConn1
  Voltage Sensor/RConn1 -- N-1/LConn1
  Lithium Cell 1RC/RConn2 -- Voltage Sensor/RConn2 -- Controlled Voltage Source/LConn1
  Lithium Cell 1RC/RConn1 -- Thermal Model/RConn1
  Lithium Cell 1RC/LConn1 -- N/LConn1
